simulink model "matching_model"  (R2018a)
settings: Solver=ode23tb  StartTime=0.0  StopTime=Tend  RelTol=1e-3
values from neighbouring files (symbols this model uses):
  C_4 = 0.1670*C_b    (= 1.00487241952e-06)    [VSM.m]    (also in dVOC.m; droop.m; droop_with_current_limitation.m; matching.m)
  C_6 = 0.2835*C_b    (= 1.70587623314e-06)    [VSM.m]    (also in dVOC.m; droop.m; droop_with_current_limitation.m; matching.m)
  C_8 = 0.2275*C_b    (= 1.36891302659e-06)    [VSM.m]    (also in dVOC.m; droop.m; droop_with_current_limitation.m; matching.m)
  C_dc = 0.008*(n)    (= 1.6)    [VSM.m]    (also in dVOC.m; droop.m; droop_with_current_limitation.m; matching.m)
  C_f = n*300*10^-6    (= 0.06)    [VSM.m]    (also in dVOC.m; droop.m; droop_with_current_limitation.m; matching.m)
  droop_percentage = 1    [VSM.m]    (also in dVOC.m; droop.m; droop_with_current_limitation.m; matching.m)
  eta_1 = w_b/Vdc_n    [VSM.m]    (also in dVOC.m; droop.m; droop_with_current_limitation.m; matching.m)
  i_ll = -1.15*(S_b/Vdc_n)-i_loss_dc    [VSM.m]    (also in dVOC.m; droop.m; droop_with_current_limitation.m; matching.m)
  i_ul = 1.15*(S_b/Vdc_n)+i_loss_dc    [VSM.m]    (also in dVOC.m; droop.m; droop_with_current_limitation.m; matching.m)
  k_dc = eta_1/(Vdc_n*m_p)    [VSM.m]    (also in dVOC.m; droop.m; droop_with_current_limitation.m; matching.m)
  K_p = (1/Vdc_n)    [VSM.m]    (also in dVOC.m; droop.m; droop_with_current_limitation.m; matching.m)
  K_r = 1/R_dc    [VSM.m]    (also in dVOC.m; droop.m; droop_with_current_limitation.m; matching.m)
  Kff_i = 1    [VSM.m]    (also in dVOC.m; droop.m; droop_with_current_limitation.m; matching.m)
  Kff_v = 1    [VSM.m]    (also in dVOC.m; droop.m; droop_with_current_limitation.m; matching.m)
  Ki_i = (1/n)*1.19    (= 0.00595)    [VSM.m]    (also in dVOC.m; droop.m; droop_with_current_limitation.m; matching.m)
  Ki_v = (n)*1.161022    (= 232.2044)    [VSM.m]    (also in dVOC.m; droop.m; droop_with_current_limitation.m; matching.m)
  ki_v_ac = 4*5.2500e-04    (= 0.0021)    [VSM.m]    (also in dVOC.m = 0.5; droop.m = 0.5; droop_with_current_limitation.m = 0.5; matching.m = 0.5)
  Kp_i = 0.738891    [VSM.m]    (also in dVOC.m; droop.m; droop_with_current_limitation.m; matching.m)
  Kp_v = 0.52    [VSM.m]    (also in dVOC.m; droop.m; droop_with_current_limitation.m; matching.m)
  kp_v_ac = 0.001    [VSM.m]    (also in dVOC.m; droop.m; droop_with_current_limitation.m; matching.m)
  L1_pu = 1*0.0186/m    (= 0.000186)    [VSM.m]    (also in dVOC.m; droop.m; droop_with_current_limitation.m; matching.m)
  L_45 = L_lines(2)    [VSM.m]    (also in dVOC.m; droop.m; droop_with_current_limitation.m; matching.m)
  L_56 = L_lines(3)    [VSM.m]    (also in dVOC.m; droop.m; droop_with_current_limitation.m; matching.m)
  L_67 = L_lines(5)    [VSM.m]    (also in dVOC.m; droop.m; droop_with_current_limitation.m; matching.m)
  L_78 = L_lines(6)    [VSM.m]    (also in dVOC.m; droop.m; droop_with_current_limitation.m; matching.m)
  L_89 = L_lines(8)    [VSM.m]    (also in dVOC.m; droop.m; droop_with_current_limitation.m; matching.m)
  L_94 = L_lines(9)    [VSM.m]    (also in dVOC.m; droop.m; droop_with_current_limitation.m; matching.m)
  L_f = (1/n)*200*10^-6    (= 1e-06)    [VSM.m]    (also in dVOC.m; droop.m; droop_with_current_limitation.m; matching.m)
  n = 200    [VSM.m]    (also in dVOC.m; droop.m; droop_with_current_limitation.m; matching.m)
  ps = base/3    (= 0.75)    [VSM.m]    (also in dVOC.m; droop.m; droop_with_current_limitation.m; matching.m)
  R1_pu = 1*0.00734/m    (= 7.34e-05)    [VSM.m]    (also in dVOC.m; droop.m; droop_with_current_limitation.m; matching.m)
  R_45 = R_lines(2)    [VSM.m]    (also in dVOC.m; droop.m; droop_with_current_limitation.m; matching.m)
  R_56 = R_lines(3)    [VSM.m]    (also in dVOC.m; droop.m; droop_with_current_limitation.m; matching.m)
  R_67 = R_lines(5)    [VSM.m]    (also in dVOC.m; droop.m; droop_with_current_limitation.m; matching.m)
  R_78 = R_lines(6)    [VSM.m]    (also in dVOC.m; droop.m; droop_with_current_limitation.m; matching.m)
  R_89 = R_lines(8)    [VSM.m]    (also in dVOC.m; droop.m; droop_with_current_limitation.m; matching.m)
  R_94 = R_lines(9)    [VSM.m]    (also in dVOC.m; droop.m; droop_with_current_limitation.m; matching.m)
  R_dc = (Vdc_n/(0.05*(S_b)/Vdc_n))    [VSM.m]    (also in dVOC.m; droop.m; droop_with_current_limitation.m; matching.m)
  R_f = 0.001/n    (= 5e-06)    [VSM.m]    (also in dVOC.m; droop.m; droop_with_current_limitation.m; matching.m)
  S_b = 100*(10^6)    (= 100000000)    [VSM.m]    (also in dVOC.m; droop.m; droop_with_current_limitation.m; matching.m)
  S_bt = S_b    (= 100000000)    [VSM.m]    (also in dVOC.m; droop.m; droop_with_current_limitation.m; matching.m)
  T_en = T_load-0.5    (= 24.5)    [VSM.m]    (also in dVOC.m; droop.m; droop_with_current_limitation.m; matching.m)
  T_load = 25    [VSM.m]    (also in dVOC.m; droop.m; droop_with_current_limitation.m; matching.m)
  T_loss = Tend    (= 50)    [dVOC.m]    (also in droop.m; droop_with_current_limitation.m)
  T_s = 1e-4    (= 0.0001)    [VSM.m]    (also in dVOC.m; droop.m; droop_with_current_limitation.m; matching.m)
  tau_dc = 0.05    [VSM.m]    (also in dVOC.m; droop.m; droop_with_current_limitation.m; matching.m)
  tau_g = 5    [VSM.m]    (also in dVOC.m; droop.m; droop_with_current_limitation.m; matching.m)
  V1_rms = 1000    [VSM.m]    (also in dVOC.m; droop.m; droop_with_current_limitation.m; matching.m)
  V2_rms = 13800    [VSM.m]    (also in dVOC.m; droop.m; droop_with_current_limitation.m; matching.m)
  V_m = sqrt(2/3)*V1_rms    [VSM.m]    (also in dVOC.m; droop.m; droop_with_current_limitation.m; matching.m)
  Vdc_n = 3*V_m    [VSM.m]    (also in dVOC.m; droop.m; droop_with_current_limitation.m; matching.m)
  w_f = 2*pi*5    (= 31.4159265359)    [VSM.m]    (also in dVOC.m; droop.m; droop_with_current_limitation.m; matching.m)
undefined symbols (not defined in the file or in its folder): D1, Delta, i_dc, k_v_ac
libraries: powerlib x88, powerlib_meascontrol x30, cstblocks x3, simulink x2, sps_avr x1
(part 2 of 2)

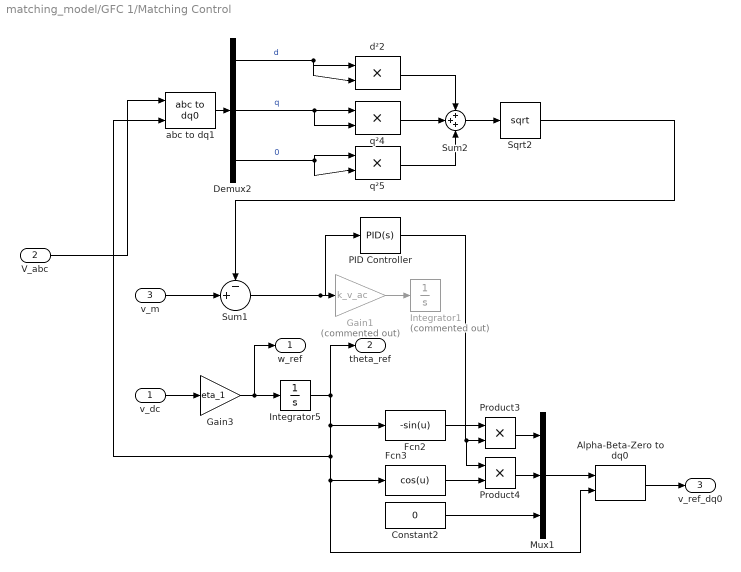
== system matching_model/GFC 1/Matching Control ==
  v_dc : Inport
  V_abc : Inport  Port=2
  v_m : Inport  Port=3
  Alpha-Beta-Zero to dq0 : powerlib_meascontrol/Transformations/Alpha-Beta-Zero to dq0  Alignment=90 degrees behind phase A axis
      settings: SourceProductName=Simscape Power Systems
  Constant2 : Constant  Value=0
  Demux2 : Demux  Outputs=3
  Fcn2 : Fcn  Expr=-sin(u)
  Fcn3 : Fcn  Expr=cos(u)
  Gain1 : Gain  Commented=on  Gain=k_v_ac
  Gain3 : Gain  Gain=eta_1
  Integrator1 : Integrator  Commented=on
  Integrator5 : Integrator
  Mux1 : Mux  Inputs=3
  PID Controller : simulink/Continuous/PID Controller  Controller=PID  TimeDomain=Continuous-time  SampleTime=-1  IntegratorMethod=Forward Euler  FilterMethod=Forward Euler  Form=Parallel  UseFilter=on  ControllerParametersSource=internal  P=kp_v_ac  I=ki_v_ac  D=0  N=100  InitialConditionSource=internal  InitialConditionForIntegrator=0  InitialConditionForFilter=0  ExternalReset=none  LimitOutput=off  UpperSaturationLimit=inf  LowerSaturationLimit=-inf  LinearizeAsGain=on  AntiWindupMode=none  Kb=1  TrackingMode=off  Kt=1  PParamMin=[]  PParamMax=[]  IParamMin=[]  IParamMax=[]  DParamMin=[]  DParamMax=[]  NParamMin=[]  NParamMax=[]  KbParamMin=[]  KbParamMax=[]  KtParamMin=[]  KtParamMax=[]  POutMin=[]  POutMax=[]  IOutMin=[]  IOutMax=[]  DOutMin=[]  DOutMax=[]  NOutMin=[]  NOutMax=[]  KbOutMin=[]  KbOutMax=[]  KtOutMin=[]  KtOutMax=[]  IntegratorOutMin=[]  IntegratorOutMax=[]  FilterOutMin=[]  FilterOutMax=[]  SumOutMin=[]  SumOutMax=[]  SumI1OutMin=[]  SumI1OutMax=[]  SumI2OutMin=[]  SumI2OutMax=[]  SumI3OutMin=[]  SumI3OutMax=[]  SumDOutMin=[]  SumDOutMax=[]  SaturationOutMin=[]  SaturationOutMax=[]  IntegratorContinuousStateAttributes=''  IntegratorStateMustResolveToSignalObject=off  IntegratorRTWStateStorageClass=Auto  FilterContinuousStateAttributes=''  FilterStateMustResolveToSignalObject=off  FilterRTWStateStorageClass=Auto  DifferentiatorICPrevScaledInput=0  DifferentiatorOutMin=[]  DifferentiatorOutMax=[]  InitialConditionSetting=State (most efficient)  FilterDiffOutCoefMin=[]  FilterDiffOutCoefMax=[]  SumDenOutMin=[]  SumDenOutMax=[]  SumNumOutMin=[]  SumNumOutMax=[]  ReciprocalOutMin=[]  ReciprocalOutMax=[]  DivideOutMin=[]  DivideOutMax=[]  TunerSelectOption=Transfer Function Based (PID Tuner App)
  Product3 : Product
  Product4 : Product
  Sqrt2 : Sqrt  SaturateOnIntegerOverflow=on
  Sum1 : Sum  Inputs=-+|
  Sum2 : Sum  Inputs=+++  SaturateOnIntegerOverflow=on  InputSameDT=on  OutDataTypeStr=Inherit: Same as first input
  abc to dq1 : powerlib_meascontrol/Transformations/abc to dq0  Alignment=90 degrees behind phase A axis
  d²2 : Product  SaturateOnIntegerOverflow=on  RndMeth=Zero  InputSameDT=on  OutDataTypeStr=Inherit: Same as first input
  q²4 : Product  SaturateOnIntegerOverflow=on  RndMeth=Zero  InputSameDT=on  OutDataTypeStr=Inherit: Same as first input
  q²5 : Product  SaturateOnIntegerOverflow=on  RndMeth=Zero  InputSameDT=on  OutDataTypeStr=Inherit: Same as first input
  w_ref : Outport
  theta_ref : Outport  Port=2
  v_ref_dq0 : Outport  Port=3
  wires:
  v_dc/1 -> Gain3/1
  Gain3/1 -> w_ref/1, Integrator5/1
  Integrator5/1 -> theta_ref/1, abc to dq1/2, Fcn3/1, Alpha-Beta-Zero to dq0/2, Fcn2/1
  Fcn2/1 -> Product3/1
  Fcn3/1 -> Product4/2
  Product3/1 -> Mux1/1
  Product4/1 -> Mux1/2
  Constant2/1 -> Mux1/3
  Mux1/1 -> Alpha-Beta-Zero to dq0/1
  v_m/1 -> Sum1/2
  Gain1/1 -> Integrator1/1
  Alpha-Beta-Zero to dq0/1 -> v_ref_dq0/1
  V_abc/1 -> abc to dq1/1
  Sqrt2/1 -> Sum1/1
  Demux2/3 -> q²5/2, q²5/1  "0"
  Sum2/1 -> Sqrt2/1
  Demux2/1 -> d²2/2, d²2/1  "d"
  q²4/1 -> Sum2/2
  d²2/1 -> Sum2/1
  Demux2/2 -> q²4/2, q²4/1  "q"
  abc to dq1/1 -> Demux2/1
  q²5/1 -> Sum2/3
  Sum1/1 -> Gain1/1, PID Controller/1
  PID Controller/1 -> Product4/1, Product3/2

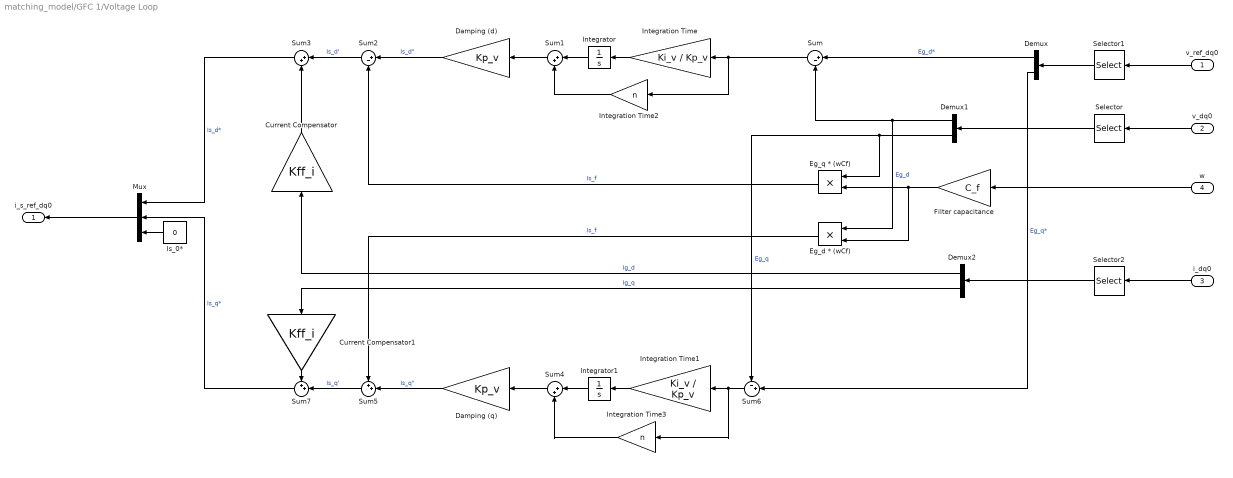
== system matching_model/GFC 1/Voltage Loop ==
  v_ref_dq0 : Inport
  v_dq0 : Inport  Port=2
  i_dq0 : Inport  Port=3
  w : Inport  Port=4
  Current Compensator : Gain  Gain=Kff_i
  Current Compensator1 : Gain  Gain=Kff_i
  Damping (d) : Gain  Gain=Kp_v
  Damping (q) : Gain  Gain=Kp_v
  Demux : Demux  Outputs=2
  Demux1 : Demux  Outputs=2
  Demux2 : Demux  Outputs=2
  Eg_d * (wCf) : Product  RndMeth=Zero
  "Eg_q * (wCf) " : Product  RndMeth=Zero
  Filter capacitance : Gain  Gain=C_f
  Integration Time : Gain  Gain=Ki_v / Kp_v
  Integration Time1 : Gain  Gain=Ki_v / Kp_v
  Integration Time2 : Gain  Gain=n
  Integration Time3 : Gain  Gain=n
  Integrator : Integrator
  Integrator1 : Integrator
  Is_0* : Constant  Value=0
  Mux : Mux  Inputs=3
  Selector : Selector  InputPortWidth=3  IndexOptions=Index vector (dialog)  Indices=[1 2]  OutputSizes=1
  Selector1 : Selector  InputPortWidth=3  IndexOptions=Index vector (dialog)  Indices=[1 2]  OutputSizes=1
  Selector2 : Selector  InputPortWidth=3  IndexOptions=Index vector (dialog)  Indices=[1 2]  OutputSizes=1
  Sum : Sum  Inputs=|+-
  Sum1 : Sum  Inputs=|++
  Sum2 : Sum  Inputs=|+-
  Sum3 : Sum  Inputs=|++
  Sum4 : Sum  Inputs=|++
  Sum5 : Sum  Inputs=++|
  Sum6 : Sum  Inputs=-+|
  Sum7 : Sum  Inputs=++|
  i_s_ref_dq0 : Outport
  wires:
  Is_0*/1 -> Mux/3
  w/1 -> Filter capacitance/1
  Integration Time1/1 -> Integrator1/1
  Integrator1/1 -> Sum4/1
  Demux/2 -> Sum6/2  "Eg_q*"
  v_ref_dq0/1 -> Selector1/1
  Eg_d * (wCf)/1 -> Sum5/1  "Is_f"
  Sum7/1 -> Mux/2  "Is_q*"
  Demux2/2 -> Current Compensator1/1  "Ig_q"
  Demux/1 -> Sum/1  "Eg_d*"
  Sum6/1 -> Integration Time3/1, Integration Time1/1
  Demux2/1 -> Current Compensator/1  "Ig_d"
  Sum2/1 -> Sum3/1  "Is_d'"
  Current Compensator/1 -> Sum3/2
  Demux1/1 -> Eg_d * (wCf)/1, Sum/2  "Eg_d"
  Current Compensator1/1 -> Sum7/1
  "Eg_q * (wCf) "/1 -> Sum2/2  "Is_f"
  Demux1/2 -> "Eg_q * (wCf) "/1, Sum6/1  "Eg_q"
  Filter capacitance/1 -> "Eg_q * (wCf) "/2, Eg_d * (wCf)/2
  Damping (d)/1 -> Sum2/1  "Is_d\""
  i_dq0/1 -> Selector2/1
  Sum5/1 -> Sum7/2  "Is_q'"
  Sum1/1 -> Damping (d)/1
  Integrator/1 -> Sum1/1
  Integration Time/1 -> Integrator/1
  Sum4/1 -> Damping (q)/1
  Sum3/1 -> Mux/1  "Is_d*"
  v_dq0/1 -> Selector/1
  Damping (q)/1 -> Sum5/2  "Is_q\""
  Selector/1 -> Demux1/1
  Selector1/1 -> Demux/1
  Selector2/1 -> Demux2/1
  Mux/1 -> i_s_ref_dq0/1
  Sum/1 -> Integration Time/1, Integration Time2/1
  Integration Time2/1 -> Sum1/2
  Integration Time3/1 -> Sum4/2

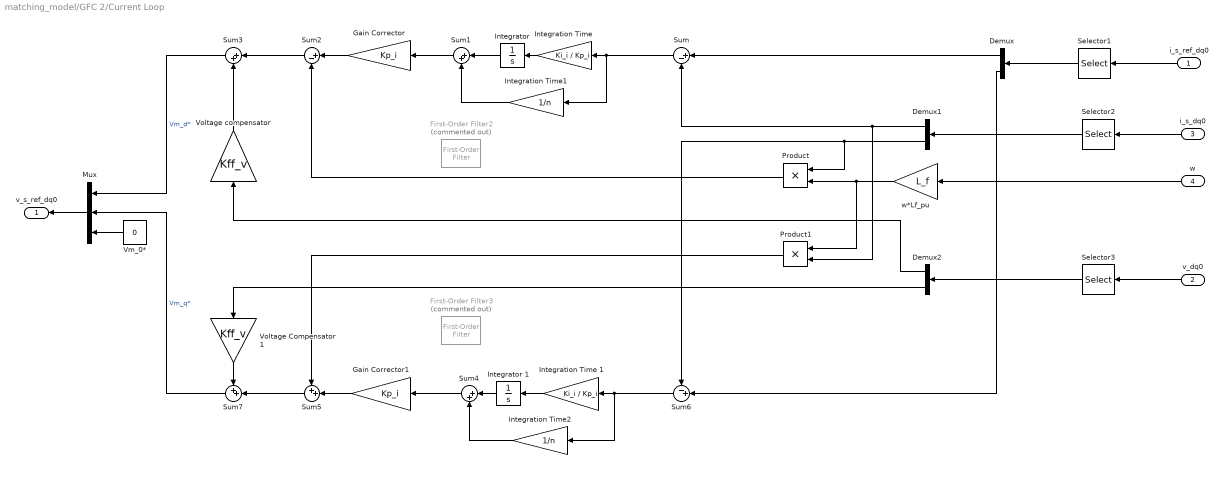
== system matching_model/GFC 2/Current Loop ==
  i_s_ref_dq0 : Inport
  v_dq0 : Inport  Port=2
  i_s_dq0 : Inport  Port=3
  w : Inport  Port=4
  Demux : Demux  Outputs=2
  Demux1 : Demux  Outputs=2
  Demux2 : Demux  Outputs=2
  First-Order Filter2 : powerlib_meascontrol/Filters/First-Order Filter  Commented=on  FilterType=Lowpass  Tc=25e-3  Ts=0  Initialize=on  Vac_Init=[0, 0, 50]  Vdc_Init=1  PlotResponse=off  FreqRange="[0,  200,  1]"
      settings: SourceProductName=Simscape Power Systems
  First-Order Filter3 : powerlib_meascontrol/Filters/First-Order Filter  Commented=on  FilterType=Lowpass  Tc=25e-3  Ts=0  Initialize=on  Vac_Init=[0, 0, 50]  Vdc_Init=0  PlotResponse=off  FreqRange="[0,  200,  1]"
      settings: SourceProductName=Simscape Power Systems
  Gain Corrector : Gain  Gain=Kp_i
  Gain Corrector1 : Gain  Gain=Kp_i
  Integration Time : Gain  Gain=Ki_i / Kp_i
  Integration Time 1 : Gain  Gain=Ki_i / Kp_i
  Integration Time1 : Gain  Gain=1/n
  Integration Time2 : Gain  Gain=1/n
  Integrator : Integrator  InitialCondition=0.0001
  Integrator 1 : Integrator
  Mux : Mux  Inputs=3
  Product : Product  RndMeth=Zero
  Product1 : Product  RndMeth=Zero
  Selector1 : Selector  InputPortWidth=3  IndexOptions=Index vector (dialog)  Indices=[1 2]  OutputSizes=1
  Selector2 : Selector  InputPortWidth=3  IndexOptions=Index vector (dialog)  Indices=[1 2]  OutputSizes=1
  Selector3 : Selector  InputPortWidth=3  IndexOptions=Index vector (dialog)  Indices=[1 2]  OutputSizes=1
  Sum : Sum  Inputs=|+-
  Sum1 : Sum  Inputs=|++
  Sum2 : Sum  Inputs=|+-
  Sum3 : Sum  Inputs=|++
  Sum4 : Sum  Inputs=|++
  Sum5 : Sum  Inputs=++|
  Sum6 : Sum  Inputs=-+|
  Sum7 : Sum  Inputs=++|
  Vm_0* : Constant  Value=0
  Voltage Compensator 1 : Gain  Gain=Kff_v
  Voltage compensator : Gain  Gain=Kff_v
  w*Lf_pu : Gain  Gain=L_f
  v_s_ref_dq0 : Outport
  wires:
  Integration Time2/1 -> Sum4/2
  Integration Time1/1 -> Sum1/2
  Gain Corrector1/1 -> Sum5/2
  Product1/1 -> Sum5/1
  Demux2/1 -> Voltage compensator/1
  Demux1/1 -> Sum/2, Product1/2
  Integrator/1 -> Sum1/1
  Vm_0*/1 -> Mux/3
  Demux1/2 -> Sum6/1, Product/1
  Selector3/1 -> Demux2/1
  i_s_dq0/1 -> Selector2/1
  Selector2/1 -> Demux1/1
  Mux/1 -> v_s_ref_dq0/1
  w/1 -> w*Lf_pu/1
  Gain Corrector/1 -> Sum2/1
  Selector1/1 -> Demux/1
  Demux/2 -> Sum6/2
  Sum4/1 -> Gain Corrector1/1
  Sum2/1 -> Sum3/1
  Sum1/1 -> Gain Corrector/1
  Voltage compensator/1 -> Sum3/2
  Integrator 1/1 -> Sum4/1
  v_dq0/1 -> Selector3/1
  i_s_ref_dq0/1 -> Selector1/1
  w*Lf_pu/1 -> Product/2, Product1/1
  Product/1 -> Sum2/2
  Voltage Compensator 1/1 -> Sum7/1
  Demux2/2 -> Voltage Compensator 1/1
  Sum7/1 -> Mux/2  "Vm_q*"
  Sum3/1 -> Mux/1  "Vm_d*"
  Demux/1 -> Sum/1
  Sum6/1 -> Integration Time2/1, Integration Time 1/1
  Sum5/1 -> Sum7/2
  Integration Time/1 -> Integrator/1
  Integration Time 1/1 -> Integrator 1/1
  Sum/1 -> Integration Time1/1, Integration Time/1

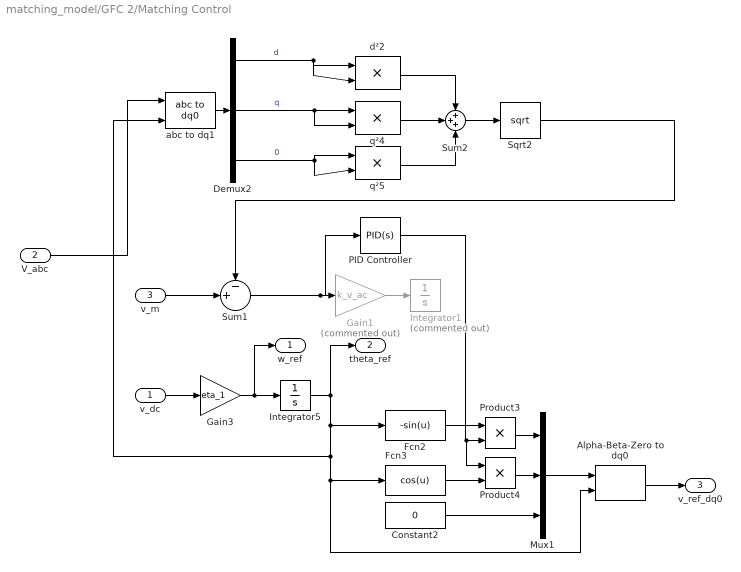
== system matching_model/GFC 2/Matching Control ==
  v_dc : Inport
  V_abc : Inport  Port=2
  v_m : Inport  Port=3
  Alpha-Beta-Zero to dq0 : powerlib_meascontrol/Transformations/Alpha-Beta-Zero to dq0  Alignment=90 degrees behind phase A axis
      settings: SourceProductName=Simscape Power Systems
  Constant2 : Constant  Value=0
  Demux2 : Demux  Outputs=3
  Fcn2 : Fcn  Expr=-sin(u)
  Fcn3 : Fcn  Expr=cos(u)
  Gain1 : Gain  Commented=on  Gain=k_v_ac
  Gain3 : Gain  Gain=eta_1
  Integrator1 : Integrator  Commented=on
  Integrator5 : Integrator
  Mux1 : Mux  Inputs=3
  PID Controller : simulink/Continuous/PID Controller  Controller=PID  TimeDomain=Continuous-time  SampleTime=-1  IntegratorMethod=Forward Euler  FilterMethod=Forward Euler  Form=Parallel  UseFilter=on  ControllerParametersSource=internal  P=kp_v_ac  I=ki_v_ac  D=0  N=100  InitialConditionSource=internal  InitialConditionForIntegrator=0  InitialConditionForFilter=0  ExternalReset=none  LimitOutput=off  UpperSaturationLimit=inf  LowerSaturationLimit=-inf  LinearizeAsGain=on  AntiWindupMode=none  Kb=1  TrackingMode=off  Kt=1  PParamMin=[]  PParamMax=[]  IParamMin=[]  IParamMax=[]  DParamMin=[]  DParamMax=[]  NParamMin=[]  NParamMax=[]  KbParamMin=[]  KbParamMax=[]  KtParamMin=[]  KtParamMax=[]  POutMin=[]  POutMax=[]  IOutMin=[]  IOutMax=[]  DOutMin=[]  DOutMax=[]  NOutMin=[]  NOutMax=[]  KbOutMin=[]  KbOutMax=[]  KtOutMin=[]  KtOutMax=[]  IntegratorOutMin=[]  IntegratorOutMax=[]  FilterOutMin=[]  FilterOutMax=[]  SumOutMin=[]  SumOutMax=[]  SumI1OutMin=[]  SumI1OutMax=[]  SumI2OutMin=[]  SumI2OutMax=[]  SumI3OutMin=[]  SumI3OutMax=[]  SumDOutMin=[]  SumDOutMax=[]  SaturationOutMin=[]  SaturationOutMax=[]  IntegratorContinuousStateAttributes=''  IntegratorStateMustResolveToSignalObject=off  IntegratorRTWStateStorageClass=Auto  FilterContinuousStateAttributes=''  FilterStateMustResolveToSignalObject=off  FilterRTWStateStorageClass=Auto  DifferentiatorICPrevScaledInput=0  DifferentiatorOutMin=[]  DifferentiatorOutMax=[]  InitialConditionSetting=State (most efficient)  FilterDiffOutCoefMin=[]  FilterDiffOutCoefMax=[]  SumDenOutMin=[]  SumDenOutMax=[]  SumNumOutMin=[]  SumNumOutMax=[]  ReciprocalOutMin=[]  ReciprocalOutMax=[]  DivideOutMin=[]  DivideOutMax=[]  TunerSelectOption=Transfer Function Based (PID Tuner App)
  Product3 : Product
  Product4 : Product
  Sqrt2 : Sqrt  SaturateOnIntegerOverflow=on
  Sum1 : Sum  Inputs=-+|
  Sum2 : Sum  Inputs=+++  SaturateOnIntegerOverflow=on  InputSameDT=on  OutDataTypeStr=Inherit: Same as first input
  abc to dq1 : powerlib_meascontrol/Transformations/abc to dq0  Alignment=90 degrees behind phase A axis
  d²2 : Product  SaturateOnIntegerOverflow=on  RndMeth=Zero  InputSameDT=on  OutDataTypeStr=Inherit: Same as first input
  q²4 : Product  SaturateOnIntegerOverflow=on  RndMeth=Zero  InputSameDT=on  OutDataTypeStr=Inherit: Same as first input
  q²5 : Product  SaturateOnIntegerOverflow=on  RndMeth=Zero  InputSameDT=on  OutDataTypeStr=Inherit: Same as first input
  w_ref : Outport
  theta_ref : Outport  Port=2
  v_ref_dq0 : Outport  Port=3
  wires:
  PID Controller/1 -> Product3/2, Product4/1
  Sum1/1 -> PID Controller/1, Gain1/1
  q²5/1 -> Sum2/3
  abc to dq1/1 -> Demux2/1
  Demux2/2 -> q²4/1, q²4/2  "q"
  d²2/1 -> Sum2/1
  q²4/1 -> Sum2/2
  Demux2/1 -> d²2/1, d²2/2  "d"
  Sum2/1 -> Sqrt2/1
  Demux2/3 -> q²5/1, q²5/2  "0"
  Sqrt2/1 -> Sum1/1
  V_abc/1 -> abc to dq1/1
  Alpha-Beta-Zero to dq0/1 -> v_ref_dq0/1
  Gain1/1 -> Integrator1/1
  v_m/1 -> Sum1/2
  Mux1/1 -> Alpha-Beta-Zero to dq0/1
  Constant2/1 -> Mux1/3
  Product4/1 -> Mux1/2
  Product3/1 -> Mux1/1
  Fcn3/1 -> Product4/2
  Fcn2/1 -> Product3/1
  Integrator5/1 -> Fcn2/1, Alpha-Beta-Zero to dq0/2, Fcn3/1, abc to dq1/2, theta_ref/1
  Gain3/1 -> Integrator5/1, w_ref/1
  v_dc/1 -> Gain3/1

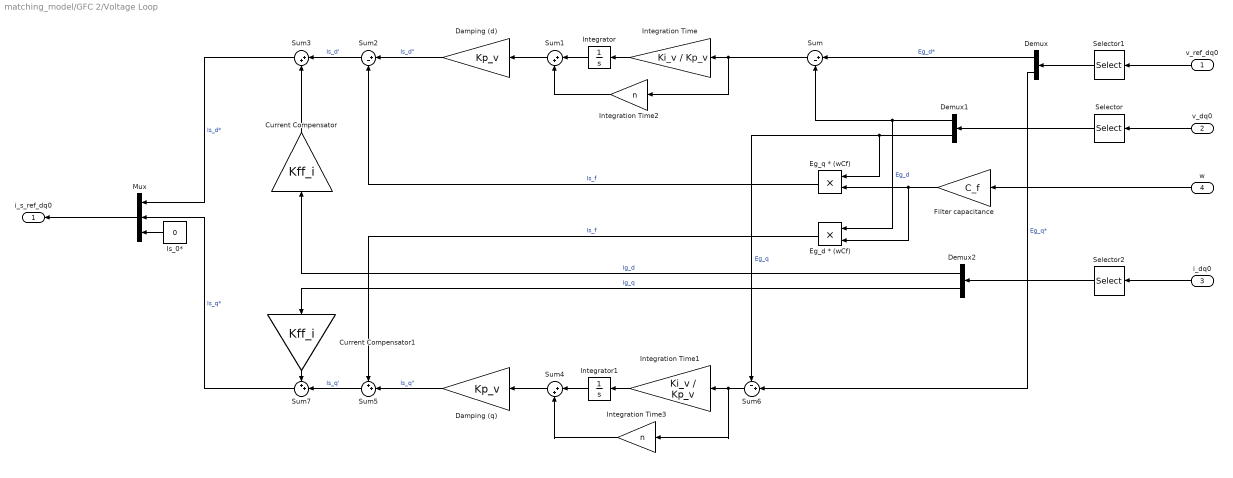
== system matching_model/GFC 2/Voltage Loop ==
  v_ref_dq0 : Inport
  v_dq0 : Inport  Port=2
  i_dq0 : Inport  Port=3
  w : Inport  Port=4
  Current Compensator : Gain  Gain=Kff_i
  Current Compensator1 : Gain  Gain=Kff_i
  Damping (d) : Gain  Gain=Kp_v
  Damping (q) : Gain  Gain=Kp_v
  Demux : Demux  Outputs=2
  Demux1 : Demux  Outputs=2
  Demux2 : Demux  Outputs=2
  Eg_d * (wCf) : Product  RndMeth=Zero
  "Eg_q * (wCf) " : Product  RndMeth=Zero
  Filter capacitance : Gain  Gain=C_f
  Integration Time : Gain  Gain=Ki_v / Kp_v
  Integration Time1 : Gain  Gain=Ki_v / Kp_v
  Integration Time2 : Gain  Gain=n
  Integration Time3 : Gain  Gain=n
  Integrator : Integrator
  Integrator1 : Integrator
  Is_0* : Constant  Value=0
  Mux : Mux  Inputs=3
  Selector : Selector  InputPortWidth=3  IndexOptions=Index vector (dialog)  Indices=[1 2]  OutputSizes=1
  Selector1 : Selector  InputPortWidth=3  IndexOptions=Index vector (dialog)  Indices=[1 2]  OutputSizes=1
  Selector2 : Selector  InputPortWidth=3  IndexOptions=Index vector (dialog)  Indices=[1 2]  OutputSizes=1
  Sum : Sum  Inputs=|+-
  Sum1 : Sum  Inputs=|++
  Sum2 : Sum  Inputs=|+-
  Sum3 : Sum  Inputs=|++
  Sum4 : Sum  Inputs=|++
  Sum5 : Sum  Inputs=++|
  Sum6 : Sum  Inputs=-+|
  Sum7 : Sum  Inputs=++|
  i_s_ref_dq0 : Outport
  wires:
  Integration Time3/1 -> Sum4/2
  Integration Time2/1 -> Sum1/2
  Sum/1 -> Integration Time2/1, Integration Time/1
  Mux/1 -> i_s_ref_dq0/1
  Selector2/1 -> Demux2/1
  Selector1/1 -> Demux/1
  Selector/1 -> Demux1/1
  Damping (q)/1 -> Sum5/2  "Is_q\""
  v_dq0/1 -> Selector/1
  Sum3/1 -> Mux/1  "Is_d*"
  Sum4/1 -> Damping (q)/1
  Integration Time/1 -> Integrator/1
  Integrator/1 -> Sum1/1
  Sum1/1 -> Damping (d)/1
  Sum5/1 -> Sum7/2  "Is_q'"
  i_dq0/1 -> Selector2/1
  Damping (d)/1 -> Sum2/1  "Is_d\""
  Filter capacitance/1 -> Eg_d * (wCf)/2, "Eg_q * (wCf) "/2
  Demux1/2 -> Sum6/1, "Eg_q * (wCf) "/1  "Eg_q"
  "Eg_q * (wCf) "/1 -> Sum2/2  "Is_f"
  Current Compensator1/1 -> Sum7/1
  Demux1/1 -> Sum/2, Eg_d * (wCf)/1  "Eg_d"
  Current Compensator/1 -> Sum3/2
  Sum2/1 -> Sum3/1  "Is_d'"
  Demux2/1 -> Current Compensator/1  "Ig_d"
  Sum6/1 -> Integration Time1/1, Integration Time3/1
  Demux/1 -> Sum/1  "Eg_d*"
  Demux2/2 -> Current Compensator1/1  "Ig_q"
  Sum7/1 -> Mux/2  "Is_q*"
  Eg_d * (wCf)/1 -> Sum5/1  "Is_f"
  v_ref_dq0/1 -> Selector1/1
  Demux/2 -> Sum6/2  "Eg_q*"
  Integrator1/1 -> Sum4/1
  Integration Time1/1 -> Integrator1/1
  w/1 -> Filter capacitance/1
  Is_0*/1 -> Mux/3

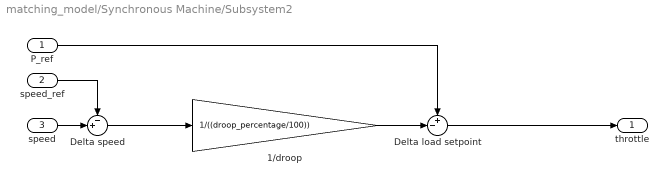
== system matching_model/Synchronous Machine/Subsystem2 ==
  P_ref : Inport
  speed_ref : Inport  Port=2
  speed : Inport  Port=3
  1/droop : Gain  Gain=1/((droop_percentage/100))
  Delta load setpoint : Sum  Inputs=+-|
  Delta speed : Sum  Inputs=-+|
  throttle : Outport
  wires:
  speed/1 -> Delta speed/2
  1/droop/1 -> Delta load setpoint/2
  Delta speed/1 -> 1/droop/1
  speed_ref/1 -> Delta speed/1
  P_ref/1 -> Delta load setpoint/1
  Delta load setpoint/1 -> throttle/1
